simulink model "SimulinkModel"  (R2023b)
settings: Solver=FixedStepAuto  StartTime=0.0  StopTime=TimeSpan  FixedStep=DT  RelTol=1e-3
values from neighbouring files (symbols this model uses):
  Amat = ABS_Amatrix(Cd,Ji,R_w,m,omega0,slope0,theta1,theta0_2,theta3,v0,wind0)    [main.m]
  AO = Amat - KO*Cmat    [main.m]
  B1mat = ABS_B1matrix(Ji)    [main.m]
  B2mat = ABS_B2matrix(Cd,Ji,R_w,m,omega0,slope0,theta1,theta0_2,theta3,v0,wind0)    [main.m]
  BO = B1mat - KO*D1mat    [main.m]
  Cemat = ABS_Cematrix(R_w,nu_v,nu_w, omega0, v0)    [main.m]
  Cmat = ABS_Cmatrix(nu_w)    [main.m]
  CO = eye(n)    [main.m]
  D1emat = ABS_D1ematrix    [main.m]
  D1mat = ABS_D1matrix    [main.m]
  D2emat = ABS_D2ematrix(R_w,nu_v,nu_w,omega0,v0)    [main.m]
  D2mat = ABS_D2matrix(omega0)    [main.m]
  DO = zeros(n, q)    [main.m]
  DT = 1e-4    (= 0.0001)    [main.m]
  e0 = 0    [main.m]
  KI = K(:, n_c+1:end)    [main.m]
  KO = Kmd.'    [main.m]
  KS = K(:, 1:n_c)    [main.m]
  lm = 1    [main.m]
  n = size(V)    [JCF.m]    (also in main.m = length(Amat))
  p = 1    [main.m]
  PLANT = 1    [main.m]
  q = length(index{i})    [JCF.m]    (also in main.m = 2)
  r = ld+q+lm    (= 8)    [main.m]    (also in reference.m = lambda_min)
  Rmat = ctrb(Amat,B1mat)    [main.m]
  u0 = tb0    [main.m]
  v_init = v0    (= 27.7777777778)    [main.m]
  w0 = [d0; nu_w; nu_v; 0]    [main.m]
  x0 = [v0; omega0; theta0_2]    [main.m]
  x_init = [v_init; omega_init; theta0_2]    [main.m]
  XOinit = x_init - x0    [main.m]
  y0 = [x0(2); x0(1)]    [main.m]
undefined symbols (not defined in the file or in its folder): rank
settings Model: Creator=nicola.mimmo2  LastModifiedBy=simon
settings DebuggingCC: UnconnectedInputMsg=warning  UnconnectedOutputMsg=warning  UnconnectedLineMsg=warning
settings ModelReferenceCC: EnableRefExpFcnMdlSchedulingChecks=on
settings RTWCC: DLArmComputeVersion=19.05

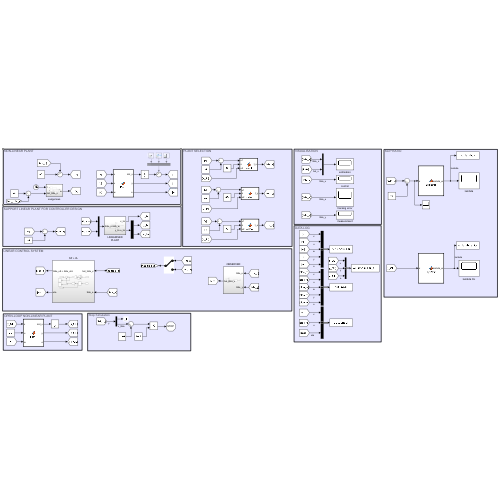
[thumbnail: Simulink's stored preview of the top-level diagram]
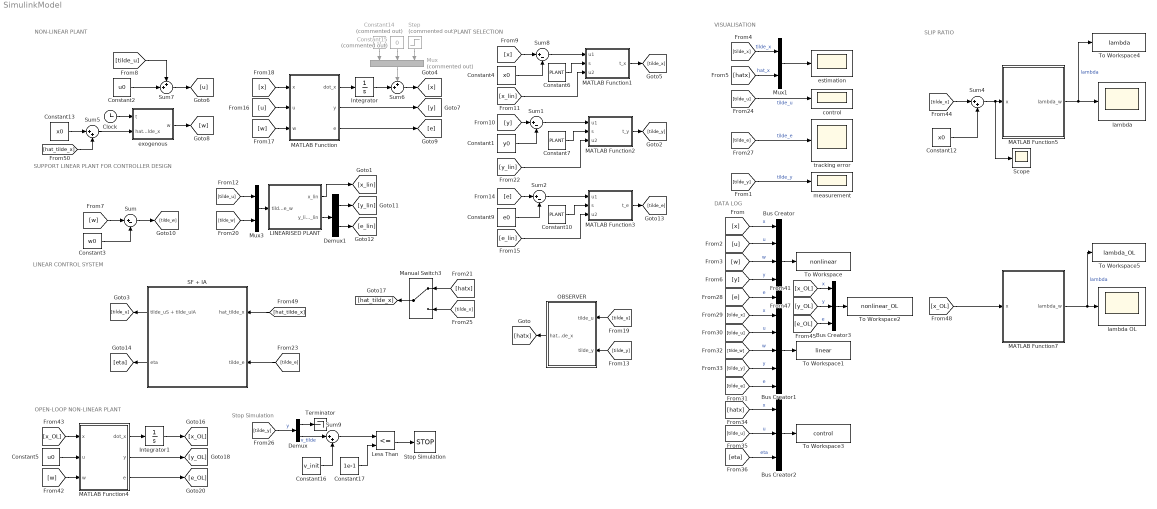
== system SimulinkModel ==
  note: Stop Simulation
  note: SLIP RATIO
  note: DATA LOG
  note: VISUALISATION
  note: PLANT SELECTION
  note: NON-LINEAR PLANT
  note: SUPPORT LINEAR PLANT FOR CONTROLLER DESIGN
  note: LINEAR CONTROL SYSTEM
  note: OPEN-LOOP NON-LINEAR PLANT
  Bus Creator : BusCreator  Inputs=5
  Bus Creator1 : BusCreator  Inputs=5
  Bus Creator2 : BusCreator  Inputs=3
  Bus Creator3 : BusCreator  Inputs=3
  Clock : Clock
  Constant1 : Constant  Value=y0
  Constant10 : Constant  Value=PLANT  VectorParams1D=off
  Constant12 : Constant  Value=x0
  Constant13 : Constant  Value=x0
  Constant14 : Constant  Commented=on  Value=0
  Constant15 : Constant  Commented=on  Value=0
  Constant16 : Constant  Value=v_init
  Constant17 : Constant  Value=1e-1
  Constant2 : Constant  Value=u0
  Constant3 : Constant  Value=w0  VectorParams1D=off
  Constant4 : Constant  Value=x0
  Constant5 : Constant  Value=u0
  Constant6 : Constant  Value=PLANT  VectorParams1D=off
  Constant7 : Constant  Value=PLANT  VectorParams1D=off
  Constant9 : Constant  Value=e0
  Demux : Demux  Outputs=2
  Demux1 : Demux  Outputs=[q lm]
  Integrator : Integrator  InitialCondition=x_init
  Integrator1 : Integrator  InitialCondition=x_init
  LINEARISED PLANT : Subsystem
  Less Than : RelationalOperator  Operator=<=  OutDataTypeStr=boolean  RndMeth=Simplest  InputSameDT=off
  MATLAB Function : MATLAB Function  TreatAsAtomicUnit=on
  MATLAB Function1 : MATLAB Function  TreatAsAtomicUnit=on
  MATLAB Function2 : MATLAB Function  TreatAsAtomicUnit=on
  MATLAB Function3 : MATLAB Function  TreatAsAtomicUnit=on
  MATLAB Function4 : MATLAB Function  TreatAsAtomicUnit=on
  MATLAB Function5 : MATLAB Function  TreatAsAtomicUnit=on
  MATLAB Function7 : MATLAB Function  TreatAsAtomicUnit=on
  Manual Switch3 : ManualSwitch
  Mux : Mux  Commented=on  Inputs=3
  Mux1 : Mux  Inputs=2
  Mux3 : Mux  Inputs=2
  OBSERVER : Subsystem
  SF + IA : Subsystem
  Scope : Scope
  Step : Step  Commented=on  After=10  SampleTime=0
  Stop Simulation : Stop
  Sum{,1..2,8} (4 alike) : Sum  Inputs=|+-
  Sum4 : Sum  Inputs=|++
  Sum5 : Sum  Inputs=|++
  Sum6 : Sum  Inputs=++|
  Sum7 : Sum  Inputs=++|
  Sum9 : Sum  Inputs=|++
  Terminator : Terminator
  To Workspace : ToWorkspace  VariableName=nonlinear  SaveFormat=Timeseries  SampleTime=-1
  To Workspace1 : ToWorkspace  VariableName=linear  SaveFormat=Timeseries  SampleTime=-1
  To Workspace2 : ToWorkspace  VariableName=nonlinear_OL  SaveFormat=Timeseries  SampleTime=-1
  To Workspace3 : ToWorkspace  VariableName=control  SaveFormat=Timeseries  SampleTime=-1
  To Workspace4 : ToWorkspace  VariableName=lambda  SaveFormat=Timeseries  SampleTime=-1
  To Workspace5 : ToWorkspace  VariableName=lambda_OL  SaveFormat=Timeseries  SampleTime=-1
  control : Scope
  estimation : Scope
  exogenous : Subsystem
  lambda : Scope
  lambda OL : Scope
  measurement : Scope
  tracking error : Scope
  wires:
  Mux3/1 -> LINEARISED PLANT/1(tilde_u tilde_w)
  OBSERVER/1(hat_tilde_x) -> [hatx]
  [tilde_x] -> Mux1/1  "tilde_x"
  [hatx] -> Mux1/2  "hat_x"
  Constant2/1 -> Sum7/2
  Sum7/1 -> [u]
  Constant1/1 -> Sum1/2
  Sum1/1 -> MATLAB Function2/1(u1)
  [y] -> Sum1/1
  [w] -> Sum/1
  [x] -> Sum8/1
  Constant4/1 -> Sum8/2
  Sum8/1 -> MATLAB Function1/1(u1)
  [tilde_e] -> SF + IA/2(tilde_e)
  [u] -> MATLAB Function/2(u)
  [w] -> MATLAB Function/3(w)
  [x] -> MATLAB Function/1(x)
  [tilde_w] -> Mux3/2
  Demux1/1 -> [y_lin]
  [tilde_u] -> OBSERVER/1(tilde_u)
  [hatx] -> Manual Switch3/1
  [tilde_x] -> Manual Switch3/2
  MATLAB Function/3(e) -> [e]
  MATLAB Function/2(y) -> [y]
  LINEARISED PLANT/1(x_lin) -> [x_lin]
  LINEARISED PLANT/2(y_lin e_lin) -> Demux1/1
  Clock/1 -> exogenous/1(t)
  MATLAB Function/1(dot_x) -> Integrator/1
  Mux1/1 -> estimation/1
  Constant6/1 -> MATLAB Function1/2(s)
  Constant7/1 -> MATLAB Function2/2(s)
  [tilde_y] -> OBSERVER/2(tilde_y)
  Constant9/1 -> Sum2/2
  Sum2/1 -> MATLAB Function3/1(u1)
  Constant10/1 -> MATLAB Function3/2(s)
  [e] -> Sum2/1
  [tilde_u] -> control/1  "tilde_u"
  [tilde_e] -> tracking error/1  "tilde_e"
  [tilde_y] -> measurement/1  "tilde_y"
  [y] -> Bus Creator/4  "y"
  [e] -> Bus Creator/5  "e"
  [w] -> Bus Creator/3  "w"
  [u] -> Bus Creator/2  "u"
  [x] -> Bus Creator/1  "x"
  Bus Creator/1 -> To Workspace/1
  [tilde_u] -> Bus Creator1/2  "u"
  [tilde_w] -> Bus Creator1/3  "w"
  [tilde_x] -> Bus Creator1/1  "x"
  [tilde_e] -> Bus Creator1/5  "e"
  [tilde_y] -> Bus Creator1/4  "y"
  Bus Creator1/1 -> To Workspace1/1
  SF + IA/2(eta) -> [eta]
  [hatx] -> Bus Creator2/1  "x"
  [tilde_u] -> Bus Creator2/2  "u"
  [eta] -> Bus Creator2/3  "eta"
  Bus Creator2/1 -> To Workspace3/1
  Integrator1/1 -> [x_OL]
  MATLAB Function4/3(e) -> [e_OL]
  MATLAB Function4/2(y) -> [y_OL]
  Constant5/1 -> MATLAB Function4/2(u)
  MATLAB Function4/1(dot_x) -> Integrator1/1
  [x_OL] -> MATLAB Function4/1(x)
  [w] -> MATLAB Function4/3(w)
  Bus Creator3/1 -> To Workspace2/1
  [x_OL] -> Bus Creator3/1  "x"
  [y_OL] -> Bus Creator3/2  "y"
  [e_OL] -> Bus Creator3/3  "e"
  MATLAB Function5/1(lambda_w) -> lambda/1, To Workspace4/1  "lambda"
  [x_OL] -> MATLAB Function7/1(x)
  MATLAB Function7/1(lambda_w) -> To Workspace5/1, lambda OL/1  "lambda"
  [x_lin] -> MATLAB Function1/3(u2)
  [y_lin] -> MATLAB Function2/3(u2)
  [e_lin] -> MATLAB Function3/3(u2)
  MATLAB Function1/1(t_x) -> [tilde_x]
  MATLAB Function2/1(t_y) -> [tilde_y]
  MATLAB Function3/1(t_e) -> [tilde_e]
  [tilde_u] -> Mux3/1
  [tilde_x] -> Sum4/1
  Sum4/1 -> Scope/1, MATLAB Function5/1(x)
  Constant12/1 -> Sum4/2
  [tilde_u] -> Sum7/1
  Demux1/2 -> [e_lin]
  Sum/1 -> [tilde_w]
  [tilde_y] -> Demux/1  "y"
  Demux/1 -> Terminator/1
  Demux/2 -> Sum9/1  "v_tilde"
  Constant16/1 -> Sum9/2
  Sum9/1 -> Less Than/1
  Constant17/1 -> Less Than/2
  Less Than/1 -> Stop Simulation/1
  [hat_tilde_x] -> SF + IA/1(hat_tilde_x)
  Manual Switch3/1 -> [hat_tilde_x]
  exogenous/1(w) -> [w]
  Constant3/1 -> Sum/2
  Constant13/1 -> Sum5/1
  [hat_tilde_x] -> Sum5/2
  Sum5/1 -> exogenous/2(hat_tilde_x)
  Sum6/1 -> [x]
  Integrator/1 -> Sum6/2
  Constant14/1 -> Mux/1
  Constant15/1 -> Mux/2
  Step/1 -> Mux/3
  Mux/1 -> Sum6/1
  SF + IA/1(tilde_uS + tilde_uIA) -> [tilde_u]

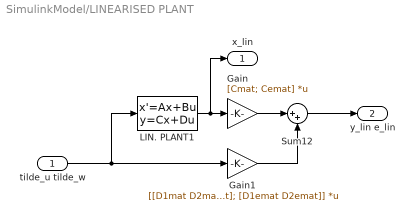
== system SimulinkModel/LINEARISED PLANT ==
  tilde_u tilde_w : Inport
  Gain : Gain  Gain=[Cmat; Cemat]  Multiplication=Matrix(K*u)
  Gain1 : Gain  Gain=[[D1mat D2mat]; [D1emat D2emat]]  Multiplication=Matrix(K*u)
  LIN. PLANT1 : StateSpace  A=Amat  B=[B1mat B2mat]  C=eye(n)  D=zeros(n,p+r)  InitialCondition=x_init-x0
  Sum12 : Sum  Inputs=|++
  x_lin : Outport
  y_lin e_lin : Outport  Port=2
  wires:
  Gain1/1 -> Sum12/2
  tilde_u tilde_w/1 -> Gain1/1, LIN. PLANT1/1
  Gain/1 -> Sum12/1
  LIN. PLANT1/1 -> x_lin/1, Gain/1
  Sum12/1 -> y_lin e_lin/1

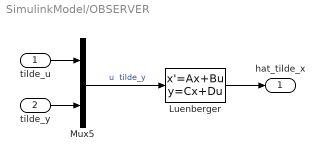
== system SimulinkModel/OBSERVER ==
  tilde_u : Inport
  tilde_y : Inport  Port=2
  Luenberger : StateSpace  A=AO  B=[BO KO]  C=CO  D=[zeros(n,p) DO]  InitialCondition=XOinit
  Mux5 : Mux  Inputs=2
  hat_tilde_x : Outport
  wires:
  tilde_u/1 -> Mux5/1
  Mux5/1 -> Luenberger/1  "u  tilde_y"
  tilde_y/1 -> Mux5/2
  Luenberger/1 -> hat_tilde_x/1

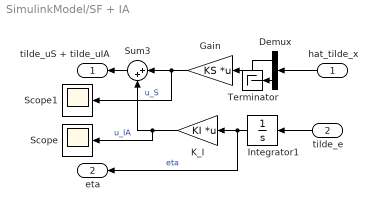
== system SimulinkModel/SF + IA ==
  hat_tilde_x : Inport
  tilde_e : Inport  Port=2
  Demux : Demux  Outputs=[rank(Rmat) (n - rank(Rmat))]
  Gain : Gain  Gain=KS  Multiplication=Matrix(K*u)
  Integrator1 : Integrator
  K_I : Gain  Gain=KI  Multiplication=Matrix(K*u)
  Scope : Scope
  Scope1 : Scope
  Sum3 : Sum  Inputs=|++
  Terminator : Terminator
  tilde_uS + tilde_uIA : Outport
  eta : Outport  Port=2
  wires:
  Gain/1 -> Scope1/1, Sum3/1  "u_S"
  Integrator1/1 -> eta/1, K_I/1  "eta"
  tilde_e/1 -> Integrator1/1
  K_I/1 -> Sum3/2, Scope/1  "u_IA"
  Sum3/1 -> tilde_uS + tilde_uIA/1
  hat_tilde_x/1 -> Demux/1
  Demux/1 -> Gain/1
  Demux/2 -> Terminator/1

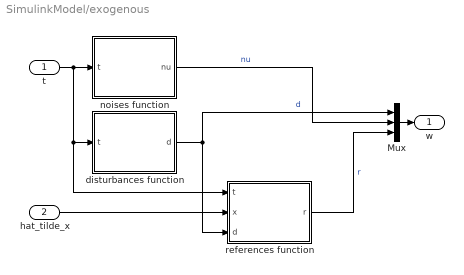
== system SimulinkModel/exogenous ==
  t : Inport
  hat_tilde_x : Inport  Port=2
  Mux : Mux  Inputs=3
  disturbances function : MATLAB Function  TreatAsAtomicUnit=on
  noises function : MATLAB Function  TreatAsAtomicUnit=on  SystemSampleTime=DT
  references function : MATLAB Function  TreatAsAtomicUnit=on
  w : Outport
  wires:
  Mux/1 -> w/1
  t/1 -> references function/1(t), disturbances function/1(t), noises function/1(t)
  disturbances function/1(d) -> Mux/1, references function/3(d)  "d"
  hat_tilde_x/1 -> references function/2(x)
  noises function/1(nu) -> Mux/2  "nu"
  references function/1(r) -> Mux/3  "r"

== matlab function SimulinkModel/MATLAB Function1 ==
  data: u1 input; s input; t_x output; u2 input
function t_x = select(u1,s,u2)

if s == 0
    t_x = u2;
else
    t_x = u1;
end

== matlab function SimulinkModel/MATLAB Function ==
  data: x input; u input; dot_x output; w input; y output; e output
function [dot_x,y,e] = Plant(x,u,w)
[dot_x,y,e] = F(x,u,w);
end

== matlab function SimulinkModel/exogenous/disturbances function ==
  data: t input; d output
function d = disturbance(t)

d = disturbance(t);

== matlab function SimulinkModel/MATLAB Function2 ==
  data: u1 input; s input; t_y output; u2 input
function t_y = select(u1,s,u2)

if s == 0
    t_y = u2;
else
    t_y = u1;
end

== matlab function SimulinkModel/exogenous/noises function ==
  data: t input; nu output
function nu = noises(t)

nu = noise(t);

== matlab function SimulinkModel/MATLAB Function3 ==
  data: u1 input; s input; t_e output; u2 input
function t_e = select(u1,s,u2)

if s == 0
    t_e = u2;
else
    t_e = u1;
end

== matlab function SimulinkModel/MATLAB Function4 ==
  data: x input; u input; dot_x output; w input; y output; e output
function [dot_x,y,e] = Plant(x,u,w)
[dot_x,y,e] = F(x,u,w);
end

== matlab function SimulinkModel/MATLAB Function5 ==
  data: x input; lambda_w output
function lambda_w = SlipRatio(x)

v = x(1);
omega = x(2);

r_w = 0.33; % [m] wheel radius
lambda_w = lambda(v,omega*r_w);

end


% slip ratio
function L = lambda(v,omegar)
if abs(v-omegar) <= 1e-4 % pure rolling / at rest
    L = 0;
else
    vmax = max(abs(v),abs(omegar));
    vmax = max(vmax,abs(omegar-v));
    L = (omegar-v)/vmax; % driving / braking
end
end

== matlab function SimulinkModel/MATLAB Function7 ==
  data: x input; lambda_w output
function lambda_w = SlipRatio(x)

v = x(1);
omega = x(2);

r_w = 0.33; % [m] wheel radius
lambda_w = lambda(v,omega*r_w);

end


% slip ratio
function L = lambda(v,omegar)
if abs(v-omegar) <= 1e-4 % pure rolling / at rest
    L = 0;
else
    vmax = max(abs(v),abs(omegar));
    vmax = max(vmax,abs(omegar-v));
    L = (omegar-v)/vmax; % driving / braking
end
end

== matlab function SimulinkModel/exogenous/references function ==
  data: t input; x input; r output; d input
function r = reference(t,x, d)
theta1 = d(1);
theta2 = x(3);
theta3 = d(2);
r = reference(t, theta1, theta2, theta3);
